simulink model "updated_target_driver_2026_withVariants"  (R2024b)
settings: Solver=FixedStepDiscrete  StartTime=0.0  StopTime=running_time  FixedStep=dt_s  RelTol=1e-3
values from neighbouring files (symbols this model uses):
  A = gamma_2*gamma_3*Thrust_desired    [force2voltage.m]
  a2_lb = -0.25    [target_driver_setup_2022_Ctrl_V_2_4.m]    (also in target_driver_setup_2022_Ctrl_V_2_4_geometric.m; target_driver_setup_mpc_12msdelay.m; target_driver_setup_mpc_andWLQP.m)
  a2_openloop = -0    (= 0)    [target_driver_setup_2022_Ctrl_V_2_4.m]    (also in target_driver_setup_2022_Ctrl_V_2_4_geometric.m = 0.6; target_driver_setup_mpc_12msdelay.m; target_driver_setup_mpc_andWLQP.m)
  a2_ub = 0.25    [target_driver_setup_2022_Ctrl_V_2_4.m]    (also in target_driver_setup_2022_Ctrl_V_2_4_geometric.m; target_driver_setup_mpc_12msdelay.m; target_driver_setup_mpc_andWLQP.m)
  adaptive_flag = 0    [target_driver_setup_2022_Ctrl_V_2_4.m]    (also in target_driver_setup_2022_Ctrl_V_2_4_geometric.m; target_driver_setup_mpc_12msdelay.m = 1; target_driver_setup_mpc_andWLQP.m = 1)
  adaptive_gain = [gamma_adaptive, adaptive_roll_limit, adaptive_pitch_limit, adaptive_yaw_limit, c_2_adaptive, gamma_lateral_adaptive, adaptive_x_limit, adaptive_y_limit, adaptive_z_limit, c_1_adaptive]    [target_driver_setup_2022_Ctrl_V_2_4.m]    (also in target_driver_setup_2022_Ctrl_V_2_4_geometric.m; target_driver_setup_mpc_12msdelay.m; target_driver_setup_mpc_andWLQP.m)
  adaptive_lateral_flag = 0    [target_driver_setup_2022_Ctrl_V_2_4.m]    (also in target_driver_setup_2022_Ctrl_V_2_4_geometric.m; target_driver_setup_mpc_12msdelay.m = 1; target_driver_setup_mpc_andWLQP.m = 1)
  adaptive_pitch_init = 0    [target_driver_setup_2022_Ctrl_V_2_4.m]    (also in target_driver_setup_2022_Ctrl_V_2_4_geometric.m; target_driver_setup_mpc_12msdelay.m; target_driver_setup_mpc_andWLQP.m)
  adaptive_pitch_limit = 0.1/(scale^2)    (= 1e-07)    [target_driver_setup_2022_Ctrl_V_2_4.m]    (also in target_driver_setup_2022_Ctrl_V_2_4_geometric.m = 3e-07; target_driver_setup_mpc_12msdelay.m; target_driver_setup_mpc_andWLQP.m)
  adaptive_pitch_limit_low = -adaptive_pitch_limit    (= -1e-07)    [target_driver_setup_2022_Ctrl_V_2_4.m]    (also in target_driver_setup_2022_Ctrl_V_2_4_geometric.m = -3e-07; target_driver_setup_mpc_12msdelay.m; target_driver_setup_mpc_andWLQP.m)
  adaptive_roll_init = 0    [target_driver_setup_2022_Ctrl_V_2_4.m]    (also in target_driver_setup_2022_Ctrl_V_2_4_geometric.m; target_driver_setup_mpc_12msdelay.m; target_driver_setup_mpc_andWLQP.m)
  adaptive_roll_limit = 0.3/(scale^2)    (= 3e-07)    [target_driver_setup_2022_Ctrl_V_2_4.m]    (also in target_driver_setup_2022_Ctrl_V_2_4_geometric.m; target_driver_setup_mpc_12msdelay.m; target_driver_setup_mpc_andWLQP.m)
  adaptive_roll_limit_low = -adaptive_roll_limit    (= -3e-07)    [target_driver_setup_2022_Ctrl_V_2_4.m]    (also in target_driver_setup_2022_Ctrl_V_2_4_geometric.m; target_driver_setup_mpc_12msdelay.m; target_driver_setup_mpc_andWLQP.m)
  adaptive_x_init = 0    [target_driver_setup_2022_Ctrl_V_2_4.m]    (also in target_driver_setup_2022_Ctrl_V_2_4_geometric.m; target_driver_setup_mpc_12msdelay.m; target_driver_setup_mpc_andWLQP.m)
  adaptive_x_limit = 0.15/(scale)    (= 0.00015)    [target_driver_setup_2022_Ctrl_V_2_4.m]    (also in target_driver_setup_2022_Ctrl_V_2_4_geometric.m = 7.5e-05; target_driver_setup_mpc_12msdelay.m; target_driver_setup_mpc_andWLQP.m)
  adaptive_x_limit_low = -adaptive_x_limit    (= -0.00015)    [target_driver_setup_2022_Ctrl_V_2_4.m]    (also in target_driver_setup_2022_Ctrl_V_2_4_geometric.m = -7.5e-05; target_driver_setup_mpc_12msdelay.m; target_driver_setup_mpc_andWLQP.m)
  adaptive_y_init = 0    [target_driver_setup_2022_Ctrl_V_2_4.m]    (also in target_driver_setup_2022_Ctrl_V_2_4_geometric.m; target_driver_setup_mpc_12msdelay.m; target_driver_setup_mpc_andWLQP.m)
  adaptive_y_limit = 0.15/(scale)    (= 0.00015)    [target_driver_setup_2022_Ctrl_V_2_4.m]    (also in target_driver_setup_2022_Ctrl_V_2_4_geometric.m = 7.5e-05; target_driver_setup_mpc_12msdelay.m; target_driver_setup_mpc_andWLQP.m)
  adaptive_y_limit_low = -adaptive_y_limit    (= -0.00015)    [target_driver_setup_2022_Ctrl_V_2_4.m]    (also in target_driver_setup_2022_Ctrl_V_2_4_geometric.m = -7.5e-05; target_driver_setup_mpc_12msdelay.m; target_driver_setup_mpc_andWLQP.m)
  adaptive_yaw_init = 0    [target_driver_setup_2022_Ctrl_V_2_4.m]    (also in target_driver_setup_2022_Ctrl_V_2_4_geometric.m; target_driver_setup_mpc_12msdelay.m; target_driver_setup_mpc_andWLQP.m)
  adaptive_yaw_limit = 0.035/(scale^2)    (= 3.5e-08)    [target_driver_setup_2022_Ctrl_V_2_4.m]    (also in target_driver_setup_2022_Ctrl_V_2_4_geometric.m; target_driver_setup_mpc_12msdelay.m; target_driver_setup_mpc_andWLQP.m)
  adaptive_yaw_limit_low = -adaptive_yaw_limit    (= -3.5e-08)    [target_driver_setup_2022_Ctrl_V_2_4.m]    (also in target_driver_setup_2022_Ctrl_V_2_4_geometric.m; target_driver_setup_mpc_12msdelay.m; target_driver_setup_mpc_andWLQP.m)
  adaptive_z_init = 0/scale    (= 0)    [target_driver_setup_2022_Ctrl_V_2_4.m]    (also in target_driver_setup_2022_Ctrl_V_2_4_geometric.m; target_driver_setup_mpc_12msdelay.m; target_driver_setup_mpc_andWLQP.m)
  adaptive_z_limit = 0.20/(scale)    (= 0.0002)    [target_driver_setup_2022_Ctrl_V_2_4.m]    (also in target_driver_setup_2022_Ctrl_V_2_4_geometric.m = 0.0008; target_driver_setup_mpc_12msdelay.m = 0.0008; target_driver_setup_mpc_andWLQP.m = 0.0008)
  adaptive_z_limit_low = -adaptive_z_limit/1    (= -0.0002)    [target_driver_setup_2022_Ctrl_V_2_4.m]    (also in target_driver_setup_2022_Ctrl_V_2_4_geometric.m = -0.0008; target_driver_setup_mpc_12msdelay.m = -0.0008; target_driver_setup_mpc_andWLQP.m = -0.0008)
  att_s = 500    [target_driver_setup_2022_Ctrl_V_2_4.m]    (also in target_driver_setup_2022_Ctrl_V_2_4_geometric.m; target_driver_setup_mpc_12msdelay.m; target_driver_setup_mpc_andWLQP.m)
  b_1_d_desired = [1,0,0]    [target_driver_setup_2022_Ctrl_V_2_4.m]    (also in target_driver_setup_2022_Ctrl_V_2_4_geometric.m; target_driver_setup_mpc_12msdelay.m; target_driver_setup_mpc_andWLQP.m)
  closedloop_flag = 1    [target_driver_setup_2022_Ctrl_V_2_4.m]    (also in target_driver_setup_2022_Ctrl_V_2_4_geometric.m = 0; target_driver_setup_mpc_12msdelay.m = 0; target_driver_setup_mpc_andWLQP.m = 0)
  control_gain = [k_x,k_v, k_R, k_Omega, k_z, k_vz, k_Rx]    [target_driver_setup_2022_Ctrl_V_2_4.m]    (also in target_driver_setup_2022_Ctrl_V_2_4_geometric.m = [k_x,k_v,k_R,k_Omega_pitch,k_Omega_roll,k_z,k_vz,k_Rx]; target_driver_setup_mpc_12msdelay.m = [k_x, k_v, k_R, k_Omega, k_z, k_vz, k_Rx,                  k; target_driver_setup_mpc_andWLQP.m = [k_x, k_v, k_R, k_Omega, k_z, k_vz, k_Rx,                  k)
  delay = delay-vicon_sample_cycle/2    [target_driver_setup_2022_Ctrl_V_2_4.m]    (also in target_driver_setup_2022_Ctrl_V_2_4_geometric.m; target_driver_setup_mpc_12msdelay.m; target_driver_setup_mpc_andWLQP.m)
  drv_amp = abs((vleft_p2p-vright_p2p))/2+min(vleft_p2p,vright_p2p)    [Wing_traj_to_Voltage.m]    (also in force2voltage.m; target_driver_setup_2022_Ctrl_V_2_4.m = 300; target_driver_setup_2022_Ctrl_V_2_4_geometric.m = 110; target_driver_setup_mpc_12msdelay.m = 150)
  drv_bias = max_drv_bias    (= 300)    [target_driver_setup_2022_Ctrl_V_2_4.m]    (also in target_driver_setup_2022_Ctrl_V_2_4_geometric.m = 200; target_driver_setup_mpc_12msdelay.m = 200; target_driver_setup_mpc_andWLQP.m = 200)
  drv_pitch_left = vleft_pitch    [Wing_traj_to_Voltage.m]    (also in force2voltage.m = 0; target_driver_setup_2022_Ctrl_V_2_4.m = 0; target_driver_setup_2022_Ctrl_V_2_4_geometric.m = 9.05; target_driver_setup_mpc_12msdelay.m = 9.05)
  drv_pitch_right = vright_pitch    [Wing_traj_to_Voltage.m]    (also in force2voltage.m = 0; target_driver_setup_2022_Ctrl_V_2_4.m = 0; target_driver_setup_2022_Ctrl_V_2_4_geometric.m = 9.05; target_driver_setup_mpc_12msdelay.m = 9.05)
  drv_roll = (vleft_p2p-vright_p2p)/4    [Wing_traj_to_Voltage.m]    (also in force2voltage.m; target_driver_setup_2022_Ctrl_V_2_4.m = 0; target_driver_setup_2022_Ctrl_V_2_4_geometric.m = -0.001; target_driver_setup_mpc_12msdelay.m = -0.001)
  dt_s = 1e-3    (= 0.001)    [target_driver_setup_2022_Ctrl_V_2_4.m]    (also in target_driver_setup_2022_Ctrl_V_2_4_geometric.m = 0.0002; target_driver_setup_mpc_12msdelay.m = 0.0002; target_driver_setup_mpc_andWLQP.m = 0.0002)
  f_fin = f    (= 180)    [target_driver_setup_2022_Ctrl_V_2_4.m]    (also in target_driver_setup_2022_Ctrl_V_2_4_geometric.m = 155; target_driver_setup_mpc_12msdelay.m = 155; target_driver_setup_mpc_andWLQP.m = 155)
  f_int = f    (= 180)    [target_driver_setup_2022_Ctrl_V_2_4.m]    (also in target_driver_setup_2022_Ctrl_V_2_4_geometric.m = 155; target_driver_setup_mpc_12msdelay.m = 155; target_driver_setup_mpc_andWLQP.m = 155)
  g = 9.8    [target_driver_setup_2022_Ctrl_V_2_4.m]    (also in target_driver_setup_2022_Ctrl_V_2_4_geometric.m; target_driver_setup_mpc_12msdelay.m; target_driver_setup_mpc_andWLQP.m = 9.81; test_full_attitude_mpc.m = 9.81)
  I_moment_vec = [Ixx, Iyy, Izz]    [target_driver_setup_2022_Ctrl_V_2_4.m]    (also in target_driver_setup_2022_Ctrl_V_2_4_geometric.m; target_driver_setup_mpc_12msdelay.m; target_driver_setup_mpc_andWLQP.m)
  landing_flag = 0    [target_driver_setup_2022_Ctrl_V_2_4.m]    (also in target_driver_setup_2022_Ctrl_V_2_4_geometric.m; target_driver_setup_mpc_12msdelay.m; target_driver_setup_mpc_andWLQP.m)
  landing_parameter = [start_delay+T,transition_rate, rising_time, falling_time, landing_rising_time, landing_z_decrease, landing_y_decrease, landing_x_decrease]    [target_driver_setup_2022_Ctrl_V_2_4.m]    (also in target_driver_setup_2022_Ctrl_V_2_4_geometric.m; target_driver_setup_mpc_12msdelay.m; target_driver_setup_mpc_andWLQP.m)
  low_bound = -8    [target_driver_setup_2022_Ctrl_V_2_4.m]    (also in target_driver_setup_2022_Ctrl_V_2_4_geometric.m = -5; target_driver_setup_mpc_12msdelay.m = -10; target_driver_setup_mpc_andWLQP.m = -10)
  low_bound_eR = -0.8    [target_driver_setup_2022_Ctrl_V_2_4.m]    (also in target_driver_setup_2022_Ctrl_V_2_4_geometric.m = -1.2; target_driver_setup_mpc_12msdelay.m = -1.2; target_driver_setup_mpc_andWLQP.m = -1.2)
  low_bound_vx = -0.5    [target_driver_setup_2022_Ctrl_V_2_4.m]    (also in target_driver_setup_2022_Ctrl_V_2_4_geometric.m; target_driver_setup_mpc_12msdelay.m; target_driver_setup_mpc_andWLQP.m)
  low_bound_vy = -0.5    [target_driver_setup_2022_Ctrl_V_2_4.m]    (also in target_driver_setup_2022_Ctrl_V_2_4_geometric.m; target_driver_setup_mpc_12msdelay.m; target_driver_setup_mpc_andWLQP.m)
  low_bound_vz = -0.5    [target_driver_setup_2022_Ctrl_V_2_4.m]    (also in target_driver_setup_2022_Ctrl_V_2_4_geometric.m; target_driver_setup_mpc_12msdelay.m; target_driver_setup_mpc_andWLQP.m)
  low_bound_x = -0.06    [target_driver_setup_2022_Ctrl_V_2_4.m]    (also in target_driver_setup_2022_Ctrl_V_2_4_geometric.m = -0.1; target_driver_setup_mpc_12msdelay.m = -0.6; target_driver_setup_mpc_andWLQP.m = -0.6)
  low_bound_y = -0.06    [target_driver_setup_2022_Ctrl_V_2_4.m]    (also in target_driver_setup_2022_Ctrl_V_2_4_geometric.m; target_driver_setup_mpc_12msdelay.m = -0.6; target_driver_setup_mpc_andWLQP.m = -0.6)
  low_bound_z = -0.04    [target_driver_setup_2022_Ctrl_V_2_4.m]    (also in target_driver_setup_2022_Ctrl_V_2_4_geometric.m; target_driver_setup_mpc_12msdelay.m = -0.1; target_driver_setup_mpc_andWLQP.m = -0.1)
  m = t <= t_zoom    [plot_roll_torque_cmd_vs_actual.m]    (also in plot_roll_torque_cmd_vs_actual_flightlog.m = t >= t0 & t <= t1; target_driver_setup_2022_Ctrl_V_2_4.m = 0.000124; target_driver_setup_2022_Ctrl_V_2_4_geometric.m = 8.5655e-05; target_driver_setup_mpc_12msdelay.m = 8.5655e-05)
  params_vec = [params_opt.delta_1, params_opt.delta_2, params_opt.delta_3,      params_opt.gamma_1, params_opt.gamma_2_1, params_opt.gamma_3,      params_opt.eta, params_opt.nu, params_opt.mu]'    [force2voltage_tuningSandbox.m]    (also in target_driver_setup_2022_Ctrl_V_2_4.m = [params_opt.delta_1, params_opt.delta_2, params_opt.delta_3,; target_driver_setup_2022_Ctrl_V_2_4_geometric.m = [params_opt.delta_1, params_opt.delta_2, params_opt.delta_3,; target_driver_setup_mpc_12msdelay.m = [params_opt.delta_1, params_opt.delta_2, params_opt.delta_3,; target_driver_setup_mpc_andWLQP.m = [params_opt.delta_1, params_opt.delta_2, params_opt.delta_3,)
  phase = 0    [target_driver_setup_2022_Ctrl_V_2_4.m]    (also in target_driver_setup_2022_Ctrl_V_2_4_geometric.m; target_driver_setup_mpc_12msdelay.m; target_driver_setup_mpc_andWLQP.m)
  r_desired = [default_x, default_y,z_desired]    [target_driver_setup_2022_Ctrl_V_2_4.m]    (also in target_driver_setup_2022_Ctrl_V_2_4_geometric.m; target_driver_setup_mpc_12msdelay.m; target_driver_setup_mpc_andWLQP.m)
  roll_offset_angle = 0    [target_driver_setup_2022_Ctrl_V_2_4.m]    (also in target_driver_setup_2022_Ctrl_V_2_4_geometric.m; target_driver_setup_mpc_12msdelay.m; target_driver_setup_mpc_andWLQP.m)
  running_time = start_delay+total_T    (= 9)    [target_driver_setup_2022_Ctrl_V_2_4.m]    (also in target_driver_setup_2022_Ctrl_V_2_4_geometric.m = 10; target_driver_setup_mpc_12msdelay.m = 0.5; target_driver_setup_mpc_andWLQP.m = 10)
  running_time_control = start_delay_control+total_T+0.0    (= 7.1)    [target_driver_setup_2022_Ctrl_V_2_4.m]    (also in target_driver_setup_2022_Ctrl_V_2_4_geometric.m = 10; target_driver_setup_mpc_12msdelay.m = 0.5; target_driver_setup_mpc_andWLQP.m = 10)
  sampling_f = 10000    [target_driver_setup_2022_Ctrl_V_2_4.m]    (also in target_driver_setup_2022_Ctrl_V_2_4_geometric.m = 5000; target_driver_setup_mpc_12msdelay.m = 5000; target_driver_setup_mpc_andWLQP.m = 5000)
  start_delay = 2.0    (= 2)    [target_driver_setup_2022_Ctrl_V_2_4.m]    (also in target_driver_setup_2022_Ctrl_V_2_4_geometric.m = 0; target_driver_setup_mpc_12msdelay.m = 0; target_driver_setup_mpc_andWLQP.m = 0)
  start_delay_control = start_delay + ramp_delay    (= 0.1)    [target_driver_setup_2022_Ctrl_V_2_4.m]    (also in target_driver_setup_2022_Ctrl_V_2_4_geometric.m = 0; target_driver_setup_mpc_12msdelay.m = 0; target_driver_setup_mpc_andWLQP.m = 0)
  T = 1    [target_driver_setup_2022_Ctrl_V_2_4.m]    (also in target_driver_setup_2022_Ctrl_V_2_4_geometric.m = 10; target_driver_setup_mpc_12msdelay.m = 0.5; target_driver_setup_mpc_andWLQP.m = 10; test_full_attitude_mpc.m = T0 + nu(1))
  task_flag = 0    [target_driver_setup_2022_Ctrl_V_2_4.m]    (also in target_driver_setup_2022_Ctrl_V_2_4_geometric.m; target_driver_setup_mpc_12msdelay.m; target_driver_setup_mpc_andWLQP.m)
  task_parameter = [radius_ref, frequency_ref, radius_ratio, lissajous_ratio, lissajous_delta, lissajous_amplitude_ratio,z_radius_ratio]    [target_driver_setup_2022_Ctrl_V_2_4.m]    (also in target_driver_setup_2022_Ctrl_V_2_4_geometric.m; target_driver_setup_mpc_12msdelay.m; target_driver_setup_mpc_andWLQP.m)
  upp_bound = 8    [target_driver_setup_2022_Ctrl_V_2_4.m]    (also in target_driver_setup_2022_Ctrl_V_2_4_geometric.m = 5; target_driver_setup_mpc_12msdelay.m = 10; target_driver_setup_mpc_andWLQP.m = 10)
  upp_bound_eR = 0.8    [target_driver_setup_2022_Ctrl_V_2_4.m]    (also in target_driver_setup_2022_Ctrl_V_2_4_geometric.m = 1.2; target_driver_setup_mpc_12msdelay.m = 1.2; target_driver_setup_mpc_andWLQP.m = 1.2)
  upp_bound_vx = 0.5    [target_driver_setup_2022_Ctrl_V_2_4.m]    (also in target_driver_setup_2022_Ctrl_V_2_4_geometric.m; target_driver_setup_mpc_12msdelay.m; target_driver_setup_mpc_andWLQP.m)
  upp_bound_vy = 0.5    [target_driver_setup_2022_Ctrl_V_2_4.m]    (also in target_driver_setup_2022_Ctrl_V_2_4_geometric.m; target_driver_setup_mpc_12msdelay.m; target_driver_setup_mpc_andWLQP.m)
  upp_bound_vz = 0.5    [target_driver_setup_2022_Ctrl_V_2_4.m]    (also in target_driver_setup_2022_Ctrl_V_2_4_geometric.m; target_driver_setup_mpc_12msdelay.m; target_driver_setup_mpc_andWLQP.m)
  upp_bound_x = 0.06    [target_driver_setup_2022_Ctrl_V_2_4.m]    (also in target_driver_setup_2022_Ctrl_V_2_4_geometric.m = 0.1; target_driver_setup_mpc_12msdelay.m = 0.6; target_driver_setup_mpc_andWLQP.m = 0.6)
  upp_bound_y = 0.06    [target_driver_setup_2022_Ctrl_V_2_4.m]    (also in target_driver_setup_2022_Ctrl_V_2_4_geometric.m; target_driver_setup_mpc_12msdelay.m = 0.6; target_driver_setup_mpc_andWLQP.m = 0.6)
  upp_bound_z = 0.04    [target_driver_setup_2022_Ctrl_V_2_4.m]    (also in target_driver_setup_2022_Ctrl_V_2_4_geometric.m; target_driver_setup_mpc_12msdelay.m = 0.1; target_driver_setup_mpc_andWLQP.m = 0.1)
undefined symbols (not defined in the file or in its folder): Com1, DiscIntNeverNeededParam, dspblkCoreblockFVToolHelper, gcbh, left_mapping, left_mapping_F_to_Phi, lp_den, lp_num, none, right_mapping, right_mapping_F_to_Phi, vlp_den, vlp_num
libraries: simulink x20, xpcseriallib x2, xpcnilib x1, xpcutilitieslib x1
(part 1 of 6)
settings Model: PacingRate=0.100000  Creator=franklinho  LastModifiedBy=franklinho
settings DebuggingCC: SignalInfNanChecking=error  UnderSpecifiedDimensionMsg=warning

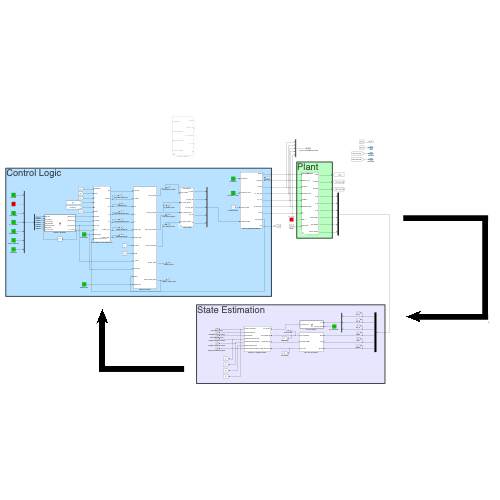
[thumbnail: Simulink's stored preview of the top-level diagram]
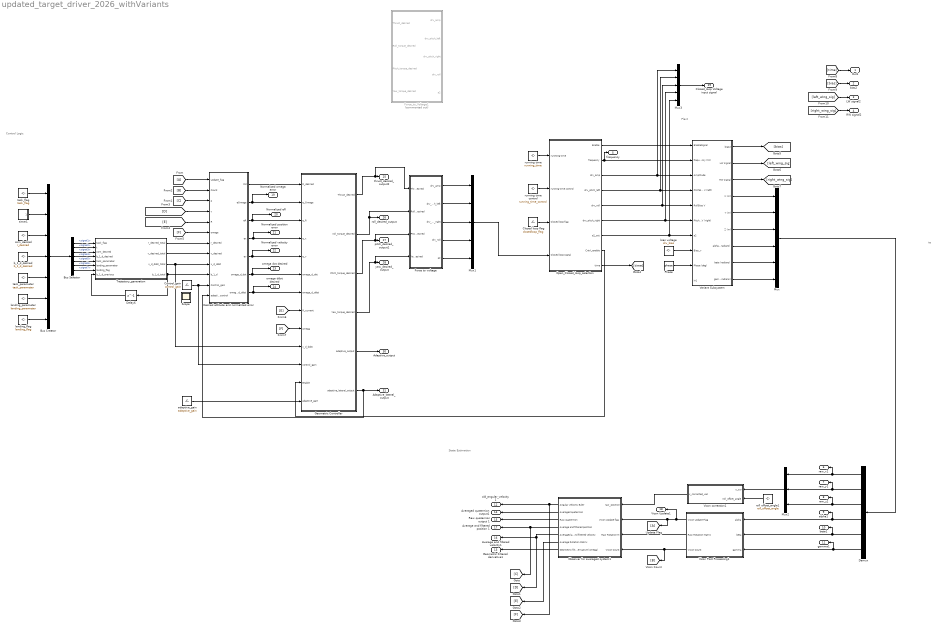
== system updated_target_driver_2026_withVariants ==
  note: te
  note: Plant
  note: State Estimation
  note: Control Logic
  Bus Creator : BusCreator  Inputs=7
  Bus Selector : BusSelector  OutputSignals=signal1,signal2,signal3,signal4,signal5,signal6,signal7
  Closed loop flag : Constant  Value=closedloop_flag
  Control_gain : Constant  Value=control_gain  SampleTime=-1
  Delay6 : Delay  DelayLength=1  InitialCondition=0
  Demux : Demux  Outputs=6
  Desired attitude and normalized error : Subsystem
  Force to voltage : Subsystem  Variant=on
  Force_to_Voltage1 : Subsystem  Commented=on
  From : From
  Geometric Controller : Subsystem
  Mux : Mux  Inputs=6
  Mux1 : Mux  Inputs=5
  Mux2 : Mux  Inputs=3
  Mux3 : Mux  Inputs=5
  Observer for averaged system1 : Subsystem
  Open_Closed_loop_selection : Subsystem
  Phase : Constant  Value=phase
  Trajectory_generation : MATLAB Function  TreatAsAtomicUnit=on
  Update Flag : Goto
  Variant Subsystem : Subsystem  Variant=on
  Vicon Post Processing1 : Subsystem
  Vicon correction1 : MATLAB Function  TreatAsAtomicUnit=on
  adaptive_gain : Constant  Value=adaptive_gain  SampleTime=-1
  b_1_d_desired : Constant  Value=b_1_d_desired  SampleTime=-1
  bias voltage : Constant  Value=drv_bias
  com_desired : Constant  Value=r_desired  SampleTime=-1
  landing_flag : Constant  Value=landing_flag  SampleTime=-1
  landing_parameter : Constant  Value=landing_parameter  SampleTime=-1
  roll_offset_angle1 : Constant  Value=roll_offset_angle  SampleTime=-1
  running time : Constant  Value=running_time  SampleTime=-1
  running time control : Constant  Value=running_time_control  SampleTime=-1
  task_flag : Constant  Value=task_flag  SampleTime=-1
  task_parameter : Constant  Value=task_parameter  SampleTime=-1
  timer1 : Subsystem
  Out1 : Outport
  bias2 : Outport  Port=2
  LW signal2 : Outport  Port=3
  RW signal2 : Outport  Port=4
  frequency : Outport  Port=5
  raw_x1 : Outport  Port=6
  raw_y1 : Outport  Port=7
  raw_z1 : Outport  Port=8
  alpha1 : Outport  Port=9
  beta1 : Outport  Port=10
  gamma1 : Outport  Port=11
  old_angular_velocity 1 : Outport  Port=12
  Geometric Filtered derivative1 : Outport  Port=13
  Averaged quaternion output1 : Outport  Port=14
  Raw quaternion output 1 : Outport  Port=15
  Average and filtered velocity1 : Outport  Port=16
  Average and filtered position 1 : Outport  Port=17
  Vicon Update1 : Outport  Port=18
  Normalized omega error : Outport  Port=19
  Normalized eR : Outport  Port=20
  Normalized position error : Outport  Port=21
  Normalized velocity error : Outport  Port=22
  omega dot desired : Outport  Port=23
  omega ddot desired : Outport  Port=24
  thrust_desired_output2 : Outport  Port=25
  roll_desired_output : Outport  Port=26
  pitch_desired_output1 : Outport  Port=27
  "yaw_desired_output " : Outport  Port=28
  Closed_loop Voltage input signal : Outport  Port=29
  Adaptive_output : Outport  Port=30
  Adaptive_lateral_output : Outport  Port=31
  Scope : Scope
  wires:
  Observer for averaged system1/1("Angular velocity Euler ") -> [F], old_angular_velocity 1/1
  Observer for averaged system1/5(Averaged and filtered velocity) -> [D], Average and filtered velocity1/1
  Observer for averaged system1/2(Averaged quaternion) -> Averaged quaternion output1/1
  Vicon Post Processing1/2(Raw Rotation Matrix) -> Observer for averaged system1/3("Raw Rotation M ")
  roll_offset_angle1/1 -> Vicon correction1/2(roll_offset_angle)
  Observer for averaged system1/4("Average and filtered position ") -> Average and filtered position 1/1, [C]
  Observer for averaged system1/3(Raw quaternion) -> Raw quaternion output 1/1
  Vicon Post Processing1/1("Vicon Update Flag ") -> Vicon Update1/1, Update Flag/1, Observer for averaged system1/2(Vicon Update flag)
  Observer for averaged system1/7(Geometric filtered derivative (omega)) -> Geometric Filtered derivative1/1
  Mux2/1 -> Vicon correction1/1(x_cur)
  Vicon Post Processing1/3("Vicon Count ") -> [B], Observer for averaged system1/4(Vicon Count)
  Vicon correction1/1(x_corrected_vec) -> Observer for averaged system1/1("raw_position ")
  Variant Subsystem/4(X (m)) -> Mux/1
  Variant Subsystem/5(Y (m)) -> Mux/2
  Variant Subsystem/6(Z (m)) -> Mux/3
  Variant Subsystem/7(alpha (radians)) -> Mux/4
  Variant Subsystem/8(beta (radians)) -> Mux/5
  Variant Subsystem/9(gamma (radians)) -> Mux/6
  Variant Subsystem/1(bias2) -> [bias]
  Variant Subsystem/2(LW signal) -> [left_wing_sig]
  Variant Subsystem/3(RW signal) -> [right_wing_sig]
  Mux/1 -> Demux/1
  Demux/1 -> raw_x1/1, Mux2/1
  Demux/3 -> raw_z1/1, Mux2/3
  Demux/2 -> raw_y1/1, Mux2/2
  Demux/4 -> alpha1/1, Vicon Post Processing1/1(alpha)
  Demux/5 -> beta1/1, Vicon Post Processing1/2(beta)
  Demux/6 -> gamma1/1, Vicon Post Processing1/3(gamma)
  running time control/1 -> Open_Closed_loop_selection/2("running time control ")
  Closed loop flag/1 -> Open_Closed_loop_selection/3(Closed loop flag)
  running time/1 -> Open_Closed_loop_selection/1(runnting time)
  Geometric Controller/2(roll_torque_desired) -> Force to voltage/2(Roll_torque_desired), roll_desired_output/1
  Geometric Controller/5(adaptive_output) -> Adaptive_output/1
  Geometric Controller/3(Pitch_torque_desired) -> Force to voltage/3(Pitch_torque_desired), pitch_desired_output1/1
  Geometric Controller/1(Thrust_desired) -> Force to voltage/1("Thrust_desired "), thrust_desired_output2/1
  Geometric Controller/4(Yaw_torque_desired) -> Force to voltage/4(Yaw_torque_desired), "yaw_desired_output "/1
  Mux1/1 -> Open_Closed_loop_selection/4(Closed loop signal)
  Open_Closed_loop_selection/1("Enable ") -> Variant Subsystem/1(EnableSignal)
  Open_Closed_loop_selection/2(frequency) -> Variant Subsystem/2(frequency (hz)), frequency/1
  Open_Closed_loop_selection/3(drv_amp) -> Mux3/1, Variant Subsystem/3(Amplitude)
  Open_Closed_loop_selection/4("drv_pitch_left ") -> Mux3/2, Variant Subsystem/4(PitchBias V (left))
  Open_Closed_loop_selection/6("drv_pitch_right ") -> Mux3/4, Variant Subsystem/6(PitchBias V (right))
  Open_Closed_loop_selection/7(a2_out) -> Mux3/5, Variant Subsystem/7(a2)
  Open_Closed_loop_selection/8(Cntrl_enable) -> Geometric Controller/12(Enable)
  Open_Closed_loop_selection/9(time) -> [time]
  bias voltage/1 -> Variant Subsystem/8(Bias_v)
  Phase/1 -> Variant Subsystem/9(Phase (deg))
  Desired attitude and normalized error/2(eOmega) -> Geometric Controller/2(e_Omega), Normalized omega error/1
  Desired attitude and normalized error/1(Rd) -> Geometric Controller/1(R_desired)
  Desired attitude and normalized error/3(eR) -> Normalized eR/1, Geometric Controller/3(e_R)
  Desired attitude and normalized error/4(ex) -> Normalized position error/1, Geometric Controller/4(e_x)
  Desired attitude and normalized error/5(ev) -> Normalized velocity error/1, Geometric Controller/5(e_v)
  Desired attitude and normalized error/6(omega_d_dot) -> omega dot desired/1, Geometric Controller/6(omega_d_dot)
  Desired attitude and normalized error/7(omega_d_ddot) -> omega ddot desired/1, Geometric Controller/7(omega_d_ddot)
  Observer for averaged system1/6(Average Rotation Matrix) -> [E]
  Trajectory_generation/1(r_desired_total) -> Desired attitude and normalized error/7(r_desired)
  Trajectory_generation/2(v_desired_total) -> Desired attitude and normalized error/8(v_desired)
  Trajectory_generation/3(x_d_ddot_total) -> Desired attitude and normalized error/9(x_d_ddot), Geometric Controller/10(x_d_ddot)
  Trajectory_generation/4(b_1_d_total) -> Delay6/1, Desired attitude and normalized error/10(b_1_d)
  Control_gain/1 -> Desired attitude and normalized error/11(Control_gain), Geometric Controller/11(control_gain)
  Geometric Controller/6(adaptive_lateral_output) -> Adaptive_lateral_output/1, Desired attitude and normalized error/12(adaptive_lateral_control)
  Mux3/1 -> Closed_loop Voltage input signal/1
  task_flag/1 -> Bus Creator/1
  timer1/1(time) -> Bus Creator/2
  com_desired/1 -> Bus Creator/3
  b_1_d_desired/1 -> Bus Creator/4
  task_parameter/1 -> Bus Creator/5
  landing_parameter/1 -> Bus Creator/6
  landing_flag/1 -> Bus Creator/7
  Bus Creator/1 -> Bus Selector/1
  Bus Selector/1 -> Trajectory_generation/1(task_flag)  "<signal1>"
  Bus Selector/2 -> Trajectory_generation/2(t)  "<signal2>"
  Bus Selector/3 -> Trajectory_generation/3(com_desired)  "<signal3>"
  Bus Selector/4 -> Trajectory_generation/4(b_1_d_desired)  "<signal4>"
  Bus Selector/5 -> Trajectory_generation/5(task_parameter)  "<signal5>"
  Bus Selector/6 -> Trajectory_generation/6(landing_parameter)  "<signal6>"
  Bus Selector/7 -> Trajectory_generation/7(landing_flag)  "<signal7>"
  Delay6/1 -> Trajectory_generation/8(b_1_d_previous)
  adaptive_gain/1 -> Geometric Controller/13(adaptive_gain)
  From/1 -> Desired attitude and normalized error/1(Update_flag)
  [B] -> Desired attitude and normalized error/2(Count)
  [C] -> Desired attitude and normalized error/3(p)
  [D] -> Desired attitude and normalized error/4(v)
  [F] -> Desired attitude and normalized error/6(omega)
  [E] -> Desired attitude and normalized error/5(R)
  [E] -> Geometric Controller/8(R_current)
  [F] -> Geometric Controller/9(omega)
  [time] -> Out1/1
  [bias] -> bias2/1
  [left_wing_sig] -> LW signal2/1
  [right_wing_sig] -> RW signal2/1
  Open_Closed_loop_selection/5("drv_roll ") -> Mux3/3, Variant Subsystem/5(RollBias V)
  Force to voltage/1(drv_amp) -> Mux1/1
  Force to voltage/2(drv_pitch_left) -> Mux1/2
  Force to voltage/3(drv_pitch_right) -> Mux1/3
  Force to voltage/4(drv_roll) -> Mux1/4
  Force to voltage/5(a2) -> Mux1/5

== system updated_target_driver_2026_withVariants/Desired attitude and normalized error ==
  Update_flag : Inport
  Count : Inport  Port=2
  p : Inport  Port=3
  v : Inport  Port=4
  R : Inport  Port=5
  omega : Inport  Port=6
  r_desired : Inport  Port=7
  v_desired : Inport  Port=8
  x_d_ddot : Inport  Port=9
  b_1_d : Inport  Port=10
  Control_gain : Inport  Port=11
  adaptive_lateral_control : Inport  Port=12
  Delay6 : Delay  DelayLength=1  InitialCondition=0
  "Desired_Attitude " : MATLAB Function  TreatAsAtomicUnit=on
  Geometric derivative for Rd in SO(3) : Subsystem
  Variant Subsystem : Subsystem  Variant=on
  m : Constant  Value=m
  m1 : Constant  Value=g
  Rd : Outport
  eOmega : Outport  Port=2
  eR : Outport  Port=3
  ex : Outport  Port=4
  ev : Outport  Port=5
  omega_d_dot : Outport  Port=6
  omega_d_ddot : Outport  Port=7
  wires:
  r_desired/1 -> Variant Subsystem/5(r_desired)
  x_d_ddot/1 -> "Desired_Attitude "/5(x_d_ddot)
  Variant Subsystem/3("Normalized position error ") -> "Desired_Attitude "/3(e_x), ex/1
  Delay6/1 -> Geometric derivative for Rd in SO(3)/1(Previous Averaged Rotation M), "Desired_Attitude "/2(R_d_prev)
  omega/1 -> Variant Subsystem/4(omega)
  "Desired_Attitude "/1(R_d_vec) -> Variant Subsystem/7(R_desired), Delay6/1, Rd/1, Geometric derivative for Rd in SO(3)/3(Current Averaged Rotation M)
  Variant Subsystem/2(Normalized eR) -> eR/1
  Count/1 -> Geometric derivative for Rd in SO(3)/2(Vicon Count)
  Update_flag/1 -> "Desired_Attitude "/10(update), Geometric derivative for Rd in SO(3)/4("Vicon Update Flag ")
  p/1 -> Variant Subsystem/1(p)
  Control_gain/1 -> "Desired_Attitude "/7(control_gain)
  v_desired/1 -> Variant Subsystem/6(v_desired)
  Geometric derivative for Rd in SO(3)/2(Filtered Geometric derivative ddRd in SO(3)1) -> omega_d_ddot/1
  v/1 -> Variant Subsystem/2(v)
  Variant Subsystem/1(Normalized omega error) -> eOmega/1
  Variant Subsystem/4(Normalized velocity error) -> "Desired_Attitude "/4(e_v), ev/1
  R/1 -> "Desired_Attitude "/1(R_cur), Variant Subsystem/3(R)
  Geometric derivative for Rd in SO(3)/1(Filtered Geometric derivative dRd in SO(3)) -> Variant Subsystem/8(omega_desired), omega_d_dot/1
  m/1 -> "Desired_Attitude "/8(m)
  m1/1 -> "Desired_Attitude "/9(g)
  b_1_d/1 -> "Desired_Attitude "/6(b_1_d)
  adaptive_lateral_control/1 -> "Desired_Attitude "/11(adaptive_lateral_control)

== system updated_target_driver_2026_withVariants/Force to voltage ==
  note: 1) Add Subsystem or Model blocks as valid variant choices.
      | 2) You cannot connect blocks at this level. At simulation, connectivity is automatically
      | determined, based on the active variant and port name matching.
  "Thrust_desired " : Inport
  Roll_torque_desired : Inport  Port=2
  Pitch_torque_desired : Inport  Port=3
  Yaw_torque_desired : Inport  Port=4
  Control Mode : Subsystem  VariantControl=replay_mode==1
  Replay Mode : Subsystem  VariantControl=replay_mode==2
  drv_amp : Outport
  drv_pitch_left : Outport  Port=2
  drv_pitch_right : Outport  Port=3
  drv_roll : Outport  Port=4
  a2 : Outport  Port=5

== system updated_target_driver_2026_withVariants/Force_to_Voltage1 ==
  note: Mapping from desired Thrust/Torque to Wing traj to Voltage mapping
      |
      | Patrick Hyun 2021 Apr
  note: a2: second-harmonic coefficient
      | Franklin Ho Jun 2026
  "Thrust_desired " : Inport
  Roll_torque_desired : Inport  Port=2
  Pitch_torque_desired : Inport  Port=3
  Yaw_torque_desired : Inport  Port=4
  A : Constant  Commented=on  Value=A
  Desired_Force_to_Voltage : MATLAB Function  TreatAsAtomicUnit=on
  "Force to Trajectory " : MATLAB Function  Commented=on  TreatAsAtomicUnit=on
  Saturation : Saturate  UpperLimit=a2_ub  LowerLimit=a2_lb
  "Trajectory to Voltage Input " : MATLAB Function  Commented=on  TreatAsAtomicUnit=on
  left_mapping : Constant  Commented=on  Value=left_mapping
  left_mapping_F_to_Phi : Constant  Commented=on  Value=left_mapping_F_to_Phi
  params_vec : Constant  Value=params_vec
  right_mapping1 : Constant  Commented=on  Value=right_mapping
  right_mapping_F_to_Phi : Constant  Commented=on  Value=right_mapping_F_to_Phi
  drv_amp : Outport
  drv_pitch_left : Outport  Port=2
  drv_pitch_right : Outport  Port=3
  drv_roll : Outport  Port=4
  a2 : Outport  Port=5
  wires:
  left_mapping/1 -> "Trajectory to Voltage Input "/4(left_mapping)
  right_mapping1/1 -> "Trajectory to Voltage Input "/5(right_mapping)
  A/1 -> "Force to Trajectory "/6(A)
  "Force to Trajectory "/1(Phi_left_p2p_desired) -> "Trajectory to Voltage Input "/1(Phi_left_p2p_command)
  "Force to Trajectory "/2(Phi_right_p2p_desired) -> "Trajectory to Voltage Input "/2(Phi_right_p2p_command)
  "Force to Trajectory "/3(Phi_pitch_desired) -> "Trajectory to Voltage Input "/3(Phi_pitch_command)
  left_mapping_F_to_Phi/1 -> "Force to Trajectory "/4(left_mapping_F_to_Phi)
  right_mapping_F_to_Phi/1 -> "Force to Trajectory "/5(right_mapping_F_to_Phi)
  Desired_Force_to_Voltage/4(drv_pitch_right) -> drv_pitch_right/1
  Desired_Force_to_Voltage/3(drv_pitch_left) -> drv_pitch_left/1
  Desired_Force_to_Voltage/2(drv_roll) -> drv_roll/1
  Desired_Force_to_Voltage/1(drv_amp) -> drv_amp/1
  "Thrust_desired "/1 -> Desired_Force_to_Voltage/1(Thrust_desired)
  Pitch_torque_desired/1 -> Desired_Force_to_Voltage/3(Pitch_torque_desired)
  Yaw_torque_desired/1 -> Desired_Force_to_Voltage/4(Yaw_torque_desired)
  params_vec/1 -> Desired_Force_to_Voltage/5(params_vec)
  Desired_Force_to_Voltage/5(a2_coeff) -> Saturation/1
  Saturation/1 -> a2/1
  Roll_torque_desired/1 -> Desired_Force_to_Voltage/2(Roll_torque_desired)

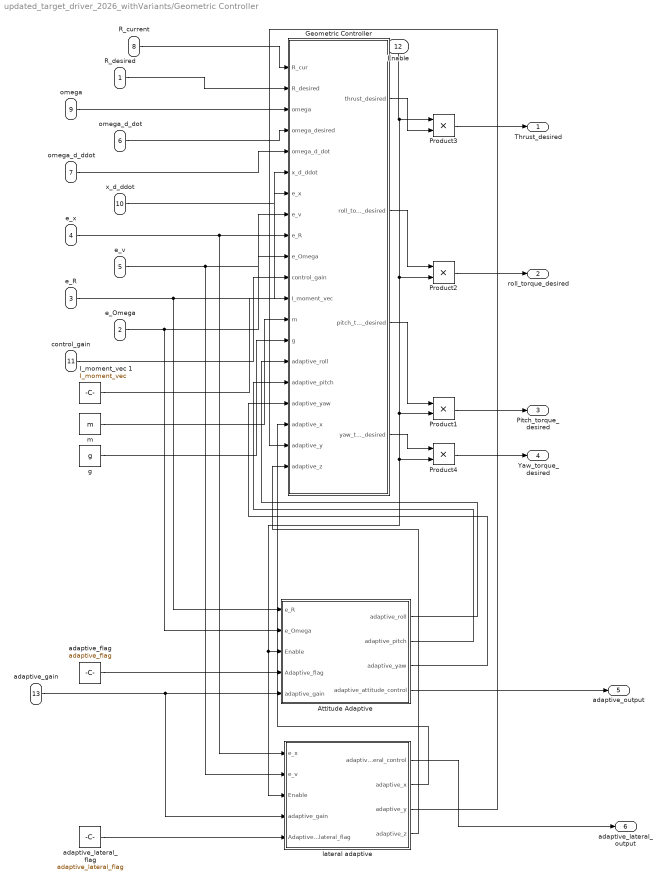
== system updated_target_driver_2026_withVariants/Geometric Controller ==
  R_desired : Inport
  e_Omega : Inport  Port=2
  e_R : Inport  Port=3
  e_x : Inport  Port=4
  e_v : Inport  Port=5
  omega_d_dot : Inport  Port=6
  omega_d_ddot : Inport  Port=7
  R_current : Inport  Port=8
  omega : Inport  Port=9
  x_d_ddot : Inport  Port=10
  control_gain : Inport  Port=11
  Enable : Inport  Port=12
  adaptive_gain : Inport  Port=13
  Attitude Adaptive : Subsystem
  Geometric Controller : MATLAB Function  TreatAsAtomicUnit=on
  I_moment_vec 1 : Constant  Value=I_moment_vec
  Product{1..4} (4 alike) : Product  RndMeth=Zero
  adaptive_flag : Constant  Value=adaptive_flag
  adaptive_lateral_flag : Constant  Value=adaptive_lateral_flag
  g : Constant  Value=g
  lateral adaptive : Subsystem
  m : Constant  Value=m
  Thrust_desired : Outport
  roll_torque_desired : Outport  Port=2
  Pitch_torque_desired : Outport  Port=3
  Yaw_torque_desired : Outport  Port=4
  adaptive_output : Outport  Port=5
  adaptive_lateral_output : Outport  Port=6
  wires:
  Product3/1 -> Thrust_desired/1
  Geometric Controller/3(pitch_torque_desired) -> Product1/1
  I_moment_vec 1/1 -> Geometric Controller/12(I_moment_vec)
  Product2/1 -> roll_torque_desired/1
  Product1/1 -> Pitch_torque_desired/1
  Geometric Controller/2(roll_torque_desired) -> Product2/1
  R_current/1 -> Geometric Controller/1(R_cur)
  Geometric Controller/1(thrust_desired) -> Product3/2
  R_desired/1 -> Geometric Controller/2(R_desired)
  omega/1 -> Geometric Controller/3(omega)
  omega_d_dot/1 -> Geometric Controller/4(omega_desired)
  omega_d_ddot/1 -> Geometric Controller/5(omega_d_dot)
  e_R/1 -> Attitude Adaptive/1(e_R), Geometric Controller/9(e_R)
  e_Omega/1 -> Attitude Adaptive/2(e_Omega), Geometric Controller/10(e_Omega)
  control_gain/1 -> Geometric Controller/11(control_gain)
  g/1 -> Geometric Controller/14(g)
  m/1 -> Geometric Controller/13(m)
  x_d_ddot/1 -> Geometric Controller/6(x_d_ddot)
  adaptive_flag/1 -> Attitude Adaptive/4(Adaptive_flag)
  adaptive_gain/1 -> lateral adaptive/4(adaptive_gain), Attitude Adaptive/5(adaptive_gain)
  Attitude Adaptive/1(adaptive_roll) -> Geometric Controller/15(adaptive_roll)
  Attitude Adaptive/2(adaptive_pitch) -> Geometric Controller/16(adaptive_pitch)
  Attitude Adaptive/3(adaptive_yaw) -> Geometric Controller/17(adaptive_yaw)
  Attitude Adaptive/4(adaptive_attitude_control) -> adaptive_output/1
  Enable/1 -> Product4/2, Attitude Adaptive/3(Enable), lateral adaptive/3(Enable), Product1/2, Product2/2, Product3/1
  Geometric Controller/4(yaw_torque_desired) -> Product4/1
  Product4/1 -> Yaw_torque_desired/1
  e_x/1 -> Geometric Controller/7(e_x), lateral adaptive/1(e_x)
  e_v/1 -> lateral adaptive/2(e_v), Geometric Controller/8(e_v)
  adaptive_lateral_flag/1 -> lateral adaptive/5(Adaptive_lateral_flag)
  lateral adaptive/1(adaptive_lateral_control) -> adaptive_lateral_output/1
  lateral adaptive/2(adaptive_x) -> Geometric Controller/18(adaptive_x)
  lateral adaptive/3(adaptive_y) -> Geometric Controller/19(adaptive_y)
  lateral adaptive/4(adaptive_z) -> Geometric Controller/20(adaptive_z)

== system updated_target_driver_2026_withVariants/Observer for averaged system1 ==
  note: Observer for averaged system using geoemtric average
      | Includes the Euler derivatives to compute the angular velocity (probably not used for control)
      | Includes the geometric average and the first order derivative in Riemannian metric SO(3)
      |
      | Patrick 2021 Mar
  "raw_position " : Inport
  Vicon Update flag : Inport  Port=2
  "Raw Rotation M " : Inport  Port=3
  Vicon Count : Inport  Port=4
  Attitude Observer : Subsystem
  "Euler derivative & filtered angular velocity " : Subsystem
  Position Observer : Subsystem
  Terminator : Terminator
  "Angular velocity Euler " : Outport
  Averaged quaternion : Outport  Port=2
  Raw quaternion : Outport  Port=3
  "Average and filtered position " : Outport  Port=4
  Averaged and filtered velocity : Outport  Port=5
  Average Rotation Matrix : Outport  Port=6
  Geometric filtered derivative (omega) : Outport  Port=7
  wires:
  "Raw Rotation M "/1 -> "Euler derivative & filtered angular velocity "/1("Rotation matrix "), Attitude Observer/2(Raw Rotation)
  Vicon Count/1 -> Attitude Observer/3(Vicon Count), Position Observer/3(Vicon Count)
  "raw_position "/1 -> Position Observer/1("raw_position ")
  Position Observer/1(Average and filtered position) -> "Average and filtered position "/1
  Position Observer/2(Averaged and filtered velocity) -> Averaged and filtered velocity/1
  "Euler derivative & filtered angular velocity "/1(Angular velocity_Euler) -> "Angular velocity Euler "/1
  Vicon Update flag/1 -> Attitude Observer/1(Vicon Update flag), Position Observer/2(vicon Update)
  Attitude Observer/1("Averaged quaternion ") -> Averaged quaternion/1
  Attitude Observer/2(Average Rotation Matrix) -> Average Rotation Matrix/1
  Attitude Observer/3(Raw quaternion) -> Raw quaternion/1
  Attitude Observer/4(Geometric filtered derivative) -> Geometric filtered derivative (omega)/1
  "Euler derivative & filtered angular velocity "/2(Frob_norm error) -> Terminator/1

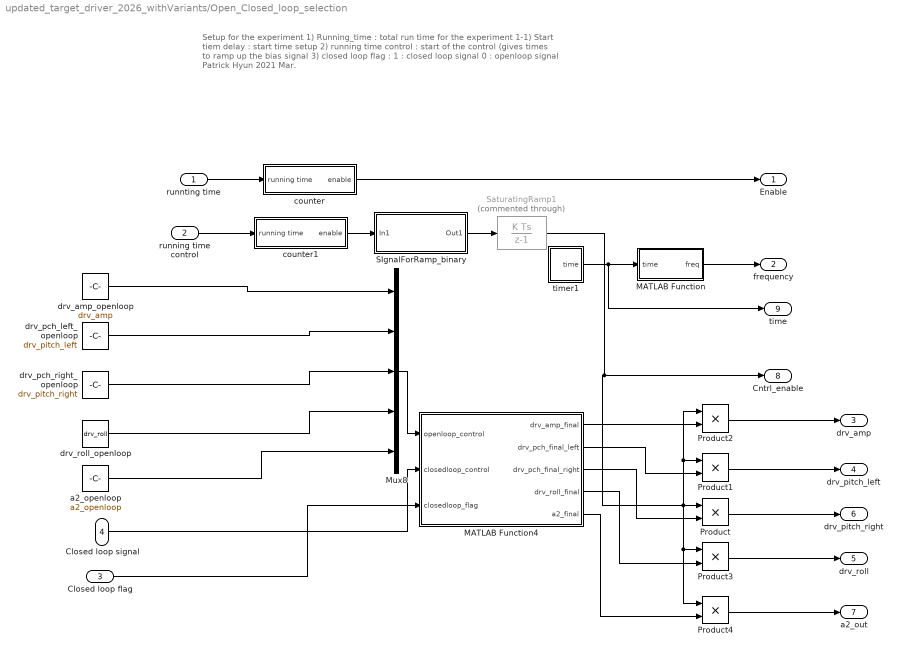
== system updated_target_driver_2026_withVariants/Open_Closed_loop_selection ==
  note: Setup for the experiment
      |
      | 1) Running_time : total run time for the experiment
      | 1-1) Start tiem delay : start time setup
      | 2) running time control : start of the control (gives times to ramp up the bias signal
      | 3) closed loop flag : 1 : closed loop signal 0 : openloop signal
      |
      | Patrick Hyun 2021 Mar.
  runnting time : Inport
  "running time control " : Inport  Port=2
  Closed loop flag : Inport  Port=3
  Closed loop signal : Inport  Port=4
  MATLAB Function : MATLAB Function  TreatAsAtomicUnit=on
  MATLAB Function4 : MATLAB Function  TreatAsAtomicUnit=on
  Mux8 : Mux  Inputs=5
  Product{,1..4} (5 alike) : Product  RndMeth=Zero
  SIgnalForRamp_binary : Subsystem
  SaturatingRamp1 : DiscreteIntegrator  Commented=through  gainval=10  SampleTime=-1  LimitOutput=on  UpperSaturationLimit=1  LowerSaturationLimit=0  ICPrevOutput=DiscIntNeverNeededParam  ICPrevScaledInput=DiscIntNeverNeededParam
  a2_openloop : Constant  Value=a2_openloop
  counter : Subsystem
  counter1 : Subsystem
  "drv_amp_openloop " : Constant  Value=drv_amp
  drv_pch_left_openloop : Constant  Value=drv_pitch_left
  drv_pch_right_openloop : Constant  Value=drv_pitch_right
  "drv_roll_openloop " : Constant  Value=drv_roll
  timer1 : Subsystem
  "Enable " : Outport
  frequency : Outport  Port=2
  drv_amp : Outport  Port=3
  "drv_pitch_left " : Outport  Port=4
  "drv_roll " : Outport  Port=5
  "drv_pitch_right " : Outport  Port=6
  a2_out : Outport  Port=7
  Cntrl_enable : Outport  Port=8
  time : Outport  Port=9
  wires:
  runnting time/1 -> counter/1(running time)
  timer1/1(time) -> time/1, MATLAB Function/1(time)
  MATLAB Function/1(freq) -> frequency/1
  SIgnalForRamp_binary/1(Out1) -> SaturatingRamp1/1
  "drv_amp_openloop "/1 -> Mux8/1
  Product1/1 -> "drv_pitch_left "/1
  counter1/1(enable) -> SIgnalForRamp_binary/1(In1)
  "running time control "/1 -> counter1/1(running time)
  Product3/1 -> "drv_roll "/1
  Closed loop flag/1 -> MATLAB Function4/3(closedloop_flag)
  MATLAB Function4/4(drv_roll_final) -> Product3/2
  Mux8/1 -> MATLAB Function4/1(openloop_control)
  MATLAB Function4/2(drv_pch_final_left) -> Product1/2
  Product2/1 -> drv_amp/1
  MATLAB Function4/1(drv_amp_final) -> Product2/2
  MATLAB Function4/3(drv_pch_final_right) -> Product/2
  Product/1 -> "drv_pitch_right "/1
  counter/1(enable) -> "Enable "/1
  Closed loop signal/1 -> MATLAB Function4/2(closedloop_control)
  Product4/1 -> a2_out/1
  MATLAB Function4/5(a2_final) -> Product4/2
  a2_openloop/1 -> Mux8/5
  SaturatingRamp1/1 -> Product4/1, Product3/1, Product2/1, Product1/1, Product/1, Cntrl_enable/1
  drv_pch_left_openloop/1 -> Mux8/2
  drv_pch_right_openloop/1 -> Mux8/3
  "drv_roll_openloop "/1 -> Mux8/4

== system updated_target_driver_2026_withVariants/Variant Subsystem ==
  note: 1) Add Subsystem or Model blocks as valid variant choices.
      | 2) You cannot connect blocks at this level. At simulation, connectivity is automatically
      | determined, based on the active variant and port name matching.
  EnableSignal : Inport
  frequency (hz) : Inport  Port=2
  Amplitude : Inport  Port=3
  PitchBias V (left) : Inport  Port=4
  RollBias V : Inport  Port=5
  PitchBias V (right) : Inport  Port=6
  a2 : Inport  Port=7
  Bias_v : Inport  Port=8
  Phase (deg) : Inport  Port=9
  In1 : Inport  Port=10
  Experimental : Subsystem  VariantControl=Plant==1
  Simulation : Subsystem  VariantControl=Plant==2
  bias2 : Outport
  LW signal : Outport  Port=2
  RW signal : Outport  Port=3
  X (m) : Outport  Port=4
  Y (m) : Outport  Port=5
  Z (m) : Outport  Port=6
  alpha (radians) : Outport  Port=7
  beta (radians) : Outport  Port=8
  gamma (radians) : Outport  Port=9

== system updated_target_driver_2026_withVariants/Vicon Post Processing1 ==
  note: Process Vicon data
      |
      | 1) Generate Raw rotation matrix
      | 2) Flag the update of new vicon data
      | 3) Count the number of samples before new update
      |
      | By Patrick 2021 Mar
  alpha : Inport
  beta : Inport  Port=2
  gamma : Inport  Port=3
  Raw rotation matrix : Subsystem
  Vicon Validity check : Subsystem
  Vicon correction : MATLAB Function  TreatAsAtomicUnit=on
  roll_offset_angle : Constant  Value=roll_offset_angle  SampleTime=-1
  "Vicon Update Flag " : Outport
  Raw Rotation Matrix : Outport  Port=2
  "Vicon Count " : Outport  Port=3
  wires:
  Vicon Validity check/2(Vicon Count) -> "Vicon Count "/1
  beta/1 -> Raw rotation matrix/2(beta)
  gamma/1 -> Raw rotation matrix/3(gamma)
  alpha/1 -> Raw rotation matrix/1(alpha)
  Vicon Validity check/1("Vicon Update flag ") -> "Vicon Update Flag "/1
  roll_offset_angle/1 -> Vicon correction/2(roll_offset_angle)
  Raw rotation matrix/1(R) -> Vicon correction/1(R_cur)
  Vicon correction/1(Rot_corrected_vec) -> Raw Rotation Matrix/1, Vicon Validity check/1("Rotation Matrix ")

== system updated_target_driver_2026_withVariants/timer1 ==
  SaturatingRamp : DiscreteIntegrator  gainval=1  SampleTime=-1  UpperSaturationLimit=1  LowerSaturationLimit=0  ICPrevOutput=DiscIntNeverNeededParam  ICPrevScaledInput=DiscIntNeverNeededParam
  constant : Constant
  time : Outport
  wires:
  SaturatingRamp/1 -> time/1
  constant/1 -> SaturatingRamp/1

== system updated_target_driver_2026_withVariants/Desired attitude and normalized error/Geometric derivative for Rd in SO(3) ==
  note: First order geometric derivative Rd in SO(3)
      | Patrick 2021 Mar
  Previous Averaged Rotation M : Inport
  Vicon Count : Inport  Port=2
  Current Averaged Rotation M : Inport  Port=3
  "Vicon Update Flag " : Inport  Port=4
  Constant : Constant  Value=sampling_f
  Demux1 : Demux  Outputs=3
  Demux2 : Demux  Outputs=3
  Discrete Derivative : simulink/Discrete/Discrete Derivative  gainval=1.0  ICPrevScaledInput=0.0  OutMin=[]  OutMax=[]  OutDataType=fixdt(1, 16)  OutScaling=2^-10  DoSatur=off
  "First order geometric derivative in SO(3) " : MATLAB Function  TreatAsAtomicUnit=on
  Mux1 : Mux  Inputs=3
  Mux2 : Mux  Inputs=3
  Previous Omega_d : Delay  DelayLength=1  InitialCondition=0
  filtered derivative1 : Subsystem
  filtered derivative5 : Subsystem
  Filtered Geometric derivative dRd in SO(3) : Outport
  Filtered Geometric derivative ddRd in SO(3)1 : Outport  Port=2
  wires:
  Previous Omega_d/1 -> "First order geometric derivative in SO(3) "/3(omega_d_prev)
  Previous Averaged Rotation M/1 -> "First order geometric derivative in SO(3) "/1(R_prev)
  Demux2/1 -> Mux2/1
  Demux2/2 -> Mux2/2
  filtered derivative5/1(Out1) -> Discrete Derivative/1, Demux2/1
  Mux2/1 -> Filtered Geometric derivative dRd in SO(3)/1
  "First order geometric derivative in SO(3) "/1(omega_d) -> filtered derivative5/1(In1), Previous Omega_d/1
  Demux2/3 -> Mux2/3
  Current Averaged Rotation M/1 -> "First order geometric derivative in SO(3) "/2(R_cur)
  Vicon Count/1 -> "First order geometric derivative in SO(3) "/5(count)
  "Vicon Update Flag "/1 -> "First order geometric derivative in SO(3) "/4(update)
  Demux1/3 -> Mux1/3
  Mux1/1 -> Filtered Geometric derivative ddRd in SO(3)1/1
  Demux1/2 -> Mux1/2
  filtered derivative1/1(Out1) -> Demux1/1
  Demux1/1 -> Mux1/1
  Discrete Derivative/1 -> filtered derivative1/1(In1)
  Constant/1 -> "First order geometric derivative in SO(3) "/6(sampling_f)

== system updated_target_driver_2026_withVariants/Desired attitude and normalized error/Variant Subsystem ==
  note: 1) Add Subsystem or Model blocks as valid variant choices.
      | 2) You cannot connect blocks at this level. At simulation, connectivity is automatically
      | determined, based on the active variant and port name matching.
  p : Inport
  v : Inport  Port=2
  R : Inport  Port=3
  omega : Inport  Port=4
  r_desired : Inport  Port=5
  v_desired : Inport  Port=6
  R_desired : Inport  Port=7
  omega_desired : Inport  Port=8
  saturated normalized error observation : Subsystem  VariantControl="controller==\"geometric\""
  unsaturated normalized error observation1 : Subsystem  VariantControl="controller==\"MPC\""
  Normalized omega error : Outport
  Normalized eR : Outport  Port=2
  "Normalized position error " : Outport  Port=3
  Normalized velocity error : Outport  Port=4

== system updated_target_driver_2026_withVariants/Force to voltage/Control Mode ==
  "Thrust_desired " : Inport
  Roll_torque_desired : Inport  Port=2
  Pitch_torque_desired : Inport  Port=3
  Yaw_torque_desired : Inport  Port=4
  Desired_Force_to_Voltage : MATLAB Function  TreatAsAtomicUnit=on
  Force_to_Voltage1 : Subsystem  Commented=on
  Saturation : Saturate  UpperLimit=a2_ub  LowerLimit=a2_lb
  params_vec : Constant  Value=params_vec
  drv_amp : Outport
  drv_pitch_left : Outport  Port=2
  drv_pitch_right : Outport  Port=3
  drv_roll : Outport  Port=4
  a2 : Outport  Port=5
  wires:
  Desired_Force_to_Voltage/5(a2_coeff) -> Saturation/1
  Yaw_torque_desired/1 -> Desired_Force_to_Voltage/4(Yaw_torque_desired)
  Roll_torque_desired/1 -> Desired_Force_to_Voltage/2(Roll_torque_desired)
  Desired_Force_to_Voltage/1(drv_amp) -> drv_amp/1
  "Thrust_desired "/1 -> Desired_Force_to_Voltage/1(Thrust_desired)
  Desired_Force_to_Voltage/3(drv_pitch_left) -> drv_pitch_left/1
  Pitch_torque_desired/1 -> Desired_Force_to_Voltage/3(Pitch_torque_desired)
  params_vec/1 -> Desired_Force_to_Voltage/5(params_vec)
  Desired_Force_to_Voltage/4(drv_pitch_right) -> drv_pitch_right/1
  Desired_Force_to_Voltage/2(drv_roll) -> drv_roll/1
  Saturation/1 -> a2/1

== system updated_target_driver_2026_withVariants/Force to voltage/Replay Mode ==
  "Thrust_desired " : Inport
  Roll_torque_desired : Inport  Port=2
  Pitch_torque_desired : Inport  Port=3
  Yaw_torque_desired : Inport  Port=4
  Demux4 : Demux
  Force_to_Voltage1 : Subsystem
  Replay commands : FromWorkspace  VariableName=robobee_load_replay_data(replay_log_file,'commands')  Interpolate=off  OutputAfterFinalValue=Holding final value
  Saturation : Saturate  UpperLimit=a2_ub  LowerLimit=a2_lb
  Term_{1..4} (4 alike) : Terminator
  drv_amp : Outport
  drv_pitch_left : Outport  Port=2
  drv_pitch_right : Outport  Port=3
  drv_roll : Outport  Port=4
  a2 : Outport  Port=5
  wires:
  Saturation/1 -> a2/1
  Force_to_Voltage1/5(a2) -> Saturation/1
  Force_to_Voltage1/4(drv_roll) -> drv_pitch_right/1
  Force_to_Voltage1/2(drv_pitch_left) -> drv_roll/1
  Force_to_Voltage1/3(drv_pitch_right) -> drv_pitch_left/1
  Force_to_Voltage1/1(drv_amp) -> drv_amp/1
  Replay commands/1 -> Demux4/1
  Demux4/1 -> Force_to_Voltage1/1("Thrust_desired ")
  Demux4/2 -> Force_to_Voltage1/2(Roll_torque_desired)
  Demux4/3 -> Force_to_Voltage1/3(Pitch_torque_desired)
  Demux4/4 -> Force_to_Voltage1/4(Yaw_torque_desired)
  "Thrust_desired "/1 -> Term_1/1
  Roll_torque_desired/1 -> Term_2/1
  Pitch_torque_desired/1 -> Term_3/1
  Yaw_torque_desired/1 -> Term_4/1
